simulink model "vestibular_system_final"  (Simulink 7.7)
settings: Solver=ode45  StartTime=0  StopTime=40  FixedStep=0.1
values from neighbouring files (symbols this model uses):
  a_lineal = get(hObject,'Value')-1    [interfaz_grafica.m]    (also in modelo_vestibular.m = 1)
  cabeza = get(hObject,'Value')-1    [interfaz_grafica.m]    (also in modelo_vestibular.m = 1)
  canal = get(hObject,'Value')-1    [interfaz_grafica.m]    (also in modelo_vestibular.m = 0)
  d = 0.76    [constantesvestibular.m]    (also in modelo_vestibular.m)
  eje_giro = get(hObject,'Value')-1    [interfaz_grafica.m]    (also in modelo_vestibular.m = 3)
  m = 1070    [constantesvestibular.m]    (also in modelo_vestibular.m)
  silla = get(hObject,'Value')-1    [interfaz_grafica.m]    (also in modelo_vestibular.m = 0)
  tau1 = 13.2    [constantesvestibular.m]    (also in modelo_vestibular.m)
  tau2 = 0.006    [constantesvestibular.m]    (also in modelo_vestibular.m)
undefined symbols (not defined in the file or in its folder): sigbuilder_block
settings Model: Creator=Ángel  LastModifiedBy=Ángel

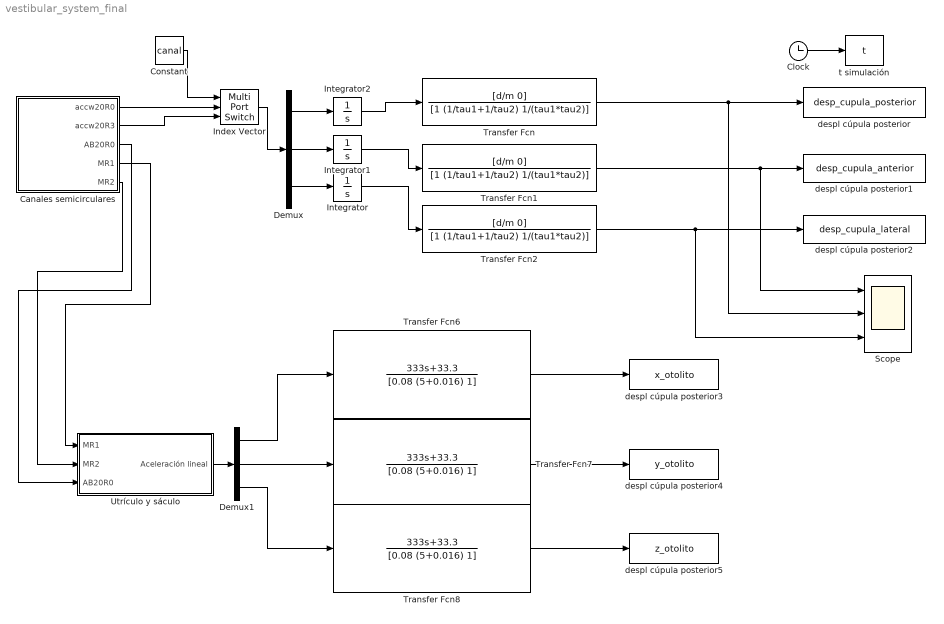
== system vestibular_system_final ==
  Canales semicirculares : Subsystem
  Clock : Clock
      settings: Decimation=10
  Constant : Constant  Value=canal
  Demux : Demux  Outputs=3
  Demux1 : Demux  Outputs=3
  Index Vector : MultiPortSwitch  DataPortOrder=Zero-based contiguous  Inputs=2  zeroidx=on
  Integrator : Integrator
  Integrator1 : Integrator
  Integrator2 : Integrator
  Scope : Scope  NumInputPorts=3
      settings: YMin=-5~-5~-5  YMax=5~5~5  SaveName=ScopeData6
  Transfer Fcn : TransferFcn  Numerator=[d/m 0]  Denominator=[1 (1/tau1+1/tau2) 1/(tau1*tau2)]
  Transfer Fcn1 : TransferFcn  Numerator=[d/m 0]  Denominator=[1 (1/tau1+1/tau2) 1/(tau1*tau2)]
  Transfer Fcn2 : TransferFcn  Numerator=[d/m 0]  Denominator=[1 (1/tau1+1/tau2) 1/(tau1*tau2)]
  Transfer Fcn6 : TransferFcn  Numerator=[333 33.3]  Denominator=[0.08 (5+0.016) 1]
  Transfer Fcn7 : TransferFcn  Numerator=[333 33.3]  Denominator=[0.08 (5+0.016) 1]
  Transfer Fcn8 : TransferFcn  Numerator=[333 33.3]  Denominator=[0.08 (5+0.016) 1]
  Utrículo y sáculo : Subsystem
  despl cúpula posterior : ToWorkspace  VariableName=desp_cupula_posterior  SampleTime=-1  SaveFormat=Array
  despl cúpula posterior1 : ToWorkspace  VariableName=desp_cupula_anterior  SampleTime=-1  SaveFormat=Array
  despl cúpula posterior2 : ToWorkspace  VariableName=desp_cupula_lateral  SampleTime=-1  SaveFormat=Array
  despl cúpula posterior3 : ToWorkspace  VariableName=x_otolito  SampleTime=-1  SaveFormat=Array
  despl cúpula posterior4 : ToWorkspace  VariableName=y_otolito  SampleTime=-1  SaveFormat=Array
  despl cúpula posterior5 : ToWorkspace  VariableName=z_otolito  SampleTime=-1  SaveFormat=Array
  t simulación : ToWorkspace  VariableName=t  SampleTime=-1  SaveFormat=Array
  wires:
  Constant/1 -> Index Vector/1
  Utrículo y sáculo/1(Aceleración lineal) -> Demux1/1
  Clock/1 -> t simulación/1
  Transfer Fcn/1 -> despl cúpula posterior/1, Scope/2
  Transfer Fcn1/1 -> despl cúpula posterior1/1, Scope/1
  Transfer Fcn2/1 -> despl cúpula posterior2/1, Scope/3
  Demux/1 -> Integrator2/1
  Demux/2 -> Integrator1/1
  Demux/3 -> Integrator/1
  Integrator2/1 -> Transfer Fcn/1
  Integrator1/1 -> Transfer Fcn1/1
  Integrator/1 -> Transfer Fcn2/1
  Canales semicirculares/1(accw20R0) -> Index Vector/2
  Canales semicirculares/2(accw20R3) -> Index Vector/3
  Canales semicirculares/3(AB20R0) -> Utrículo y sáculo/3(AB20R0)
  Canales semicirculares/4(MR1) -> Utrículo y sáculo/1(MR1)
  Canales semicirculares/5(MR2) -> Utrículo y sáculo/2(MR2)
  Index Vector/1 -> Demux/1
  Demux1/1 -> Transfer Fcn6/1
  Demux1/2 -> Transfer Fcn7/1
  Demux1/3 -> Transfer Fcn8/1
  Transfer Fcn6/1 -> despl cúpula posterior3/1
  Transfer Fcn7/1 -> despl cúpula posterior4/1
  Transfer Fcn8/1 -> despl cúpula posterior5/1

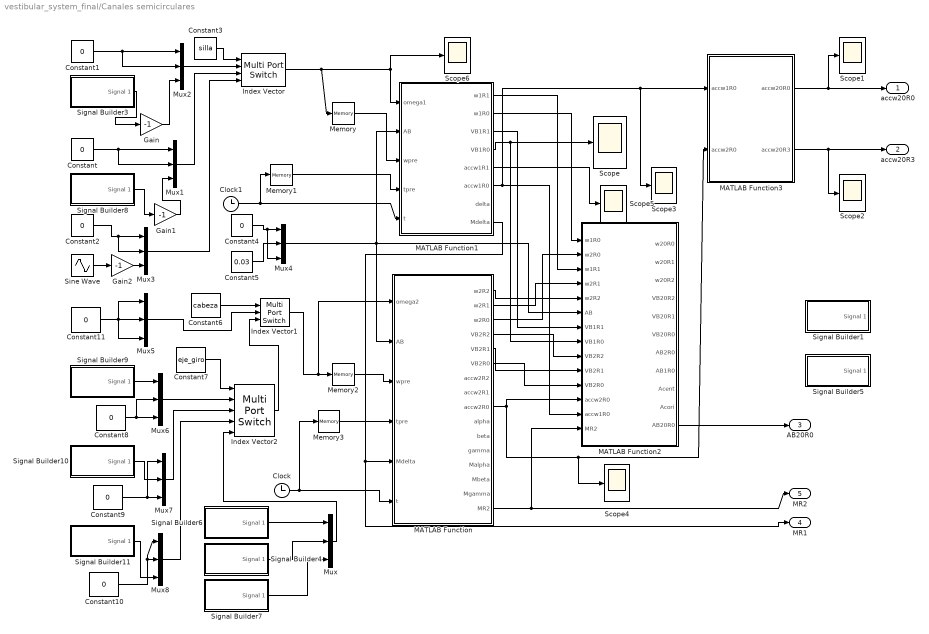
== system vestibular_system_final/Canales semicirculares ==
  Clock : Clock
      settings: Decimation=10
  Clock1 : Clock
      settings: Decimation=10
  Constant{,1..2,4,8..11} (8 alike) : Constant  Value=0
  Constant3 : Constant  Value=silla
  Constant5 : Constant  Value=0.03
  Constant6 : Constant  Value=cabeza
  Constant7 : Constant  Value=eje_giro
  Gain : Gain  Gain=-1
  Gain1 : Gain  Gain=-1
  Gain2 : Gain  Gain=-1
  Index Vector : MultiPortSwitch  DataPortOrder=Zero-based contiguous  zeroidx=on
  Index Vector1 : MultiPortSwitch  DataPortOrder=Zero-based contiguous  Inputs=2  zeroidx=on
  Index Vector2 : MultiPortSwitch  DataPortOrder=Zero-based contiguous  Inputs=4  zeroidx=on
  MATLAB Function : Stateflow chart  TreatAsAtomicUnit=on
  MATLAB Function1 : Stateflow chart  TreatAsAtomicUnit=on
  MATLAB Function2 : Stateflow chart  TreatAsAtomicUnit=on
  MATLAB Function3 : Stateflow chart  TreatAsAtomicUnit=on
  Memory{,1..3} (4 alike) : Memory
  Mux{,1..8} (9 alike) : Mux  Inputs=3
  Scope{,1..6} (7 alike) : Scope
      Scope2 settings: SaveName=ScopeData2
      Scope3 settings: SaveName=ScopeData3
      Scope4 settings: SaveName=ScopeData4
      Scope5 settings: TimeRange=40  YMin=0  YMax=0.16  SaveName=ScopeData7
      Scope6 settings: SaveName=ScopeData8
  Signal Builder1 : Subsystem  Tag=STV Subsys  LoadFcn=sigbuilder_block('load');  StartFcn=sigbuilder_block('start');  StopFcn=sigbuilder_block('stop');  ClipboardFcn=sigbuilder_block('clipboard');  mask(Sigbuilder block){}
      mask help: Create and generate interchangeable groups of signals whose waveforms are piecewise linear.
      mask init:
      | if ~strcmp(get_param(bdroot(gcbh),'SimulationStatus'),'stopped') tuvar = sigbuilder_block('maskInit'); end
      settings: CopyFcn=sigbuilder_block('copy');  DeleteFcn=sigbuilder_block('delete');  ModelCloseFcn=sigbuilder_block('modelClose');  PreSaveFcn=sigbuilder_block('preSave');  NameChangeFcn=sigbuilder_block('namechange');  OpenFcn=sigbuilder_block('open',[437.25 118.5 550.5 394.5 ]);  CloseFcn=sigbuilder_block('close');
      mask Display: plot(0, 0, 100, 100,[2, 2, 32, 32, 2], [68, 8, 8, 68, 68],[32, 2], [38, 38], [32, 19, 2],[53, 60, 44], [32, 17, 17, 2],[16, 16, 31, 31]);txt = getActiveGroup(gcbh);text(2, 100, txt,'verticalAlignment', 'top');
  Signal Builder10 : Subsystem  Tag=STV Subsys  LoadFcn=sigbuilder_block('load');  StartFcn=sigbuilder_block('start');  StopFcn=sigbuilder_block('stop');  ClipboardFcn=sigbuilder_block('clipboard');  mask(Sigbuilder block){}
      mask help: Create and generate interchangeable groups of signals whose waveforms are piecewise linear.
      mask init:
      | if ~strcmp(get_param(bdroot(gcbh),'SimulationStatus'),'stopped') tuvar = sigbuilder_block('maskInit'); end
      settings: CopyFcn=sigbuilder_block('copy');  DeleteFcn=sigbuilder_block('delete');  ModelCloseFcn=sigbuilder_block('modelClose');  PreSaveFcn=sigbuilder_block('preSave');  NameChangeFcn=sigbuilder_block('namechange');  OpenFcn=sigbuilder_block('open',[437.25 118.5 550.5 394.5 ]);  CloseFcn=sigbuilder_block('close');
      mask Display: plot(0, 0, 100, 100,[2, 2, 32, 32, 2], [68, 8, 8, 68, 68],[32, 2], [38, 38], [32, 19, 2],[53, 60, 44], [32, 17, 17, 2],[16, 16, 31, 31]);txt = getActiveGroup(gcbh);text(2, 100, txt,'verticalAlignment', 'top');
  Signal Builder11 : Subsystem  Tag=STV Subsys  LoadFcn=sigbuilder_block('load');  StartFcn=sigbuilder_block('start');  StopFcn=sigbuilder_block('stop');  ClipboardFcn=sigbuilder_block('clipboard');  mask(Sigbuilder block){}
      mask help: Create and generate interchangeable groups of signals whose waveforms are piecewise linear.
      mask init:
      | if ~strcmp(get_param(bdroot(gcbh),'SimulationStatus'),'stopped') tuvar = sigbuilder_block('maskInit'); end
      settings: CopyFcn=sigbuilder_block('copy');  DeleteFcn=sigbuilder_block('delete');  ModelCloseFcn=sigbuilder_block('modelClose');  PreSaveFcn=sigbuilder_block('preSave');  NameChangeFcn=sigbuilder_block('namechange');  OpenFcn=sigbuilder_block('open',[437.25 118.5 550.5 394.5 ]);  CloseFcn=sigbuilder_block('close');
      mask Display: plot(0, 0, 100, 100,[2, 2, 32, 32, 2], [68, 8, 8, 68, 68],[32, 2], [38, 38], [32, 19, 2],[53, 60, 44], [32, 17, 17, 2],[16, 16, 31, 31]);txt = getActiveGroup(gcbh);text(2, 100, txt,'verticalAlignment', 'top');
  Signal Builder3 : Subsystem  Tag=STV Subsys  LoadFcn=sigbuilder_block('load');  StartFcn=sigbuilder_block('start');  StopFcn=sigbuilder_block('stop');  ClipboardFcn=sigbuilder_block('clipboard');  mask(Sigbuilder block){}
      mask help: Create and generate interchangeable groups of signals whose waveforms are piecewise linear.
      mask init:
      | if ~strcmp(get_param(bdroot(gcbh),'SimulationStatus'),'stopped') tuvar = sigbuilder_block('maskInit'); end
      settings: CopyFcn=sigbuilder_block('copy');  DeleteFcn=sigbuilder_block('delete');  ModelCloseFcn=sigbuilder_block('modelClose');  PreSaveFcn=sigbuilder_block('preSave');  NameChangeFcn=sigbuilder_block('namechange');  OpenFcn=sigbuilder_block('open',[437.25 118.5 550.5 394.5 ]);  CloseFcn=sigbuilder_block('close');
      mask Display: plot(0, 0, 100, 100,[2, 2, 32, 32, 2], [68, 8, 8, 68, 68],[32, 2], [38, 38], [32, 19, 2],[53, 60, 44], [32, 17, 17, 2],[16, 16, 31, 31]);txt = getActiveGroup(gcbh);text(2, 100, txt,'verticalAlignment', 'top');
  Signal Builder4 : Subsystem  Tag=STV Subsys  LoadFcn=sigbuilder_block('load');  StartFcn=sigbuilder_block('start');  StopFcn=sigbuilder_block('stop');  ClipboardFcn=sigbuilder_block('clipboard');  mask(Sigbuilder block){}
      mask help: Create and generate interchangeable groups of signals whose waveforms are piecewise linear.
      mask init:
      | if ~strcmp(get_param(bdroot(gcbh),'SimulationStatus'),'stopped') tuvar = sigbuilder_block('maskInit'); end
      settings: CopyFcn=sigbuilder_block('copy');  DeleteFcn=sigbuilder_block('delete');  ModelCloseFcn=sigbuilder_block('modelClose');  PreSaveFcn=sigbuilder_block('preSave');  NameChangeFcn=sigbuilder_block('namechange');  OpenFcn=sigbuilder_block('open',[437.25 118.5 550.5 394.5 ]);  CloseFcn=sigbuilder_block('close');
      mask Display: plot(0, 0, 100, 100,[2, 2, 32, 32, 2], [68, 8, 8, 68, 68],[32, 2], [38, 38], [32, 19, 2],[53, 60, 44], [32, 17, 17, 2],[16, 16, 31, 31]);txt = getActiveGroup(gcbh);text(2, 100, txt,'verticalAlignment', 'top');
  Signal Builder5 : Subsystem  Tag=STV Subsys  LoadFcn=sigbuilder_block('load');  StartFcn=sigbuilder_block('start');  StopFcn=sigbuilder_block('stop');  ClipboardFcn=sigbuilder_block('clipboard');  mask(Sigbuilder block){}
      mask help: Create and generate interchangeable groups of signals whose waveforms are piecewise linear.
      mask init:
      | if ~strcmp(get_param(bdroot(gcbh),'SimulationStatus'),'stopped') tuvar = sigbuilder_block('maskInit'); end
      settings: CopyFcn=sigbuilder_block('copy');  DeleteFcn=sigbuilder_block('delete');  ModelCloseFcn=sigbuilder_block('modelClose');  PreSaveFcn=sigbuilder_block('preSave');  NameChangeFcn=sigbuilder_block('namechange');  OpenFcn=sigbuilder_block('open',[437.25 118.5 550.5 394.5 ]);  CloseFcn=sigbuilder_block('close');
      mask Display: plot(0, 0, 100, 100,[2, 2, 32, 32, 2], [68, 8, 8, 68, 68],[32, 2], [38, 38], [32, 19, 2],[53, 60, 44], [32, 17, 17, 2],[16, 16, 31, 31]);txt = getActiveGroup(gcbh);text(2, 100, txt,'verticalAlignment', 'top');
  Signal Builder6 : Subsystem  Tag=STV Subsys  LoadFcn=sigbuilder_block('load');  StartFcn=sigbuilder_block('start');  StopFcn=sigbuilder_block('stop');  ClipboardFcn=sigbuilder_block('clipboard');  mask(Sigbuilder block){}
      mask help: Create and generate interchangeable groups of signals whose waveforms are piecewise linear.
      mask init:
      | if ~strcmp(get_param(bdroot(gcbh),'SimulationStatus'),'stopped') tuvar = sigbuilder_block('maskInit'); end
      settings: CopyFcn=sigbuilder_block('copy');  DeleteFcn=sigbuilder_block('delete');  ModelCloseFcn=sigbuilder_block('modelClose');  PreSaveFcn=sigbuilder_block('preSave');  NameChangeFcn=sigbuilder_block('namechange');  OpenFcn=sigbuilder_block('open',[437.25 118.5 550.5 394.5 ]);  CloseFcn=sigbuilder_block('close');
      mask Display: plot(0, 0, 100, 100,[2, 2, 32, 32, 2], [68, 8, 8, 68, 68],[32, 2], [38, 38], [32, 19, 2],[53, 60, 44], [32, 17, 17, 2],[16, 16, 31, 31]);txt = getActiveGroup(gcbh);text(2, 100, txt,'verticalAlignment', 'top');
  Signal Builder7 : Subsystem  Tag=STV Subsys  LoadFcn=sigbuilder_block('load');  StartFcn=sigbuilder_block('start');  StopFcn=sigbuilder_block('stop');  ClipboardFcn=sigbuilder_block('clipboard');  mask(Sigbuilder block){}
      mask help: Create and generate interchangeable groups of signals whose waveforms are piecewise linear.
      mask init:
      | if ~strcmp(get_param(bdroot(gcbh),'SimulationStatus'),'stopped') tuvar = sigbuilder_block('maskInit'); end
      settings: CopyFcn=sigbuilder_block('copy');  DeleteFcn=sigbuilder_block('delete');  ModelCloseFcn=sigbuilder_block('modelClose');  PreSaveFcn=sigbuilder_block('preSave');  NameChangeFcn=sigbuilder_block('namechange');  OpenFcn=sigbuilder_block('open',[437.25 118.5 550.5 394.5 ]);  CloseFcn=sigbuilder_block('close');
      mask Display: plot(0, 0, 100, 100,[2, 2, 32, 32, 2], [68, 8, 8, 68, 68],[32, 2], [38, 38], [32, 19, 2],[53, 60, 44], [32, 17, 17, 2],[16, 16, 31, 31]);txt = getActiveGroup(gcbh);text(2, 100, txt,'verticalAlignment', 'top');
  Signal Builder8 : Subsystem  Tag=STV Subsys  LoadFcn=sigbuilder_block('load');  StartFcn=sigbuilder_block('start');  StopFcn=sigbuilder_block('stop');  ClipboardFcn=sigbuilder_block('clipboard');  mask(Sigbuilder block){}
      mask help: Create and generate interchangeable groups of signals whose waveforms are piecewise linear.
      mask init:
      | if ~strcmp(get_param(bdroot(gcbh),'SimulationStatus'),'stopped') tuvar = sigbuilder_block('maskInit'); end
      settings: CopyFcn=sigbuilder_block('copy');  DeleteFcn=sigbuilder_block('delete');  ModelCloseFcn=sigbuilder_block('modelClose');  PreSaveFcn=sigbuilder_block('preSave');  NameChangeFcn=sigbuilder_block('namechange');  OpenFcn=sigbuilder_block('open',[437.25 118.5 550.5 394.5 ]);  CloseFcn=sigbuilder_block('close');
      mask Display: plot(0, 0, 100, 100,[2, 2, 32, 32, 2], [68, 8, 8, 68, 68],[32, 2], [38, 38], [32, 19, 2],[53, 60, 44], [32, 17, 17, 2],[16, 16, 31, 31]);txt = getActiveGroup(gcbh);text(2, 100, txt,'verticalAlignment', 'top');
  Signal Builder9 : Subsystem  Tag=STV Subsys  LoadFcn=sigbuilder_block('load');  StartFcn=sigbuilder_block('start');  StopFcn=sigbuilder_block('stop');  ClipboardFcn=sigbuilder_block('clipboard');  mask(Sigbuilder block){}
      mask help: Create and generate interchangeable groups of signals whose waveforms are piecewise linear.
      mask init:
      | if ~strcmp(get_param(bdroot(gcbh),'SimulationStatus'),'stopped') tuvar = sigbuilder_block('maskInit'); end
      settings: CopyFcn=sigbuilder_block('copy');  DeleteFcn=sigbuilder_block('delete');  ModelCloseFcn=sigbuilder_block('modelClose');  PreSaveFcn=sigbuilder_block('preSave');  NameChangeFcn=sigbuilder_block('namechange');  OpenFcn=sigbuilder_block('open',[437.25 118.5 550.5 394.5 ]);  CloseFcn=sigbuilder_block('close');
      mask Display: plot(0, 0, 100, 100,[2, 2, 32, 32, 2], [68, 8, 8, 68, 68],[32, 2], [38, 38], [32, 19, 2],[53, 60, 44], [32, 17, 17, 2],[16, 16, 31, 31]);txt = getActiveGroup(gcbh);text(2, 100, txt,'verticalAlignment', 'top');
  Sine Wave : Sin  Amplitude=1.7453  Frequency=0.5  SampleTime=0
  accw20R0 : Outport
  accw20R3 : Outport  Port=2
  AB20R0 : Outport  Port=3
  MR1 : Outport  Port=4
  MR2 : Outport  Port=5
  wires:
  MATLAB Function/16(MR2) -> MATLAB Function2/14(MR2), MR2/1
  Clock/1 -> Memory3/1, MATLAB Function/6(t)
  Constant/1 -> Mux1/1, Mux1/2
  Constant1/1 -> Mux2/1, Mux2/2
  Constant2/1 -> Mux3/1, Mux3/2
  Constant3/1 -> Index Vector/1
  Mux3/1 -> Index Vector/4
  Constant4/1 -> Mux4/1, Mux4/3
  Constant5/1 -> Mux4/2
  Mux4/1 -> MATLAB Function1/2(AB), MATLAB Function/2(AB), MATLAB Function2/6(AB)
  Index Vector/1 -> Memory/1, MATLAB Function1/1(omega1), Scope6/1
  Clock1/1 -> MATLAB Function1/5(t), Memory1/1
  MATLAB Function1/4(VB1R0) -> Scope/1, MATLAB Function2/8(VB1R0)
  MATLAB Function1/8(Mdelta) -> MATLAB Function/5(Mdelta), MR1/1
  MATLAB Function/3(w2R0) -> MATLAB Function2/2(w2R0)
  MATLAB Function1/2(w1R0) -> MATLAB Function2/1(w1R0)
  MATLAB Function1/1(w1R1) -> MATLAB Function2/3(w1R1)
  MATLAB Function/2(w2R1) -> MATLAB Function2/4(w2R1)
  MATLAB Function/1(w2R2) -> MATLAB Function2/5(w2R2)
  MATLAB Function/4(VB2R2) -> MATLAB Function2/9(VB2R2)
  MATLAB Function/5(VB2R1) -> MATLAB Function2/10(VB2R1)
  MATLAB Function/6(VB2R0) -> MATLAB Function2/11(VB2R0)
  MATLAB Function1/3(VB1R1) -> MATLAB Function2/7(VB1R1)
  MATLAB Function1/6(accw1R0) -> MATLAB Function3/1(accw1R0), Scope3/1, MATLAB Function2/13(accw1R0)
  MATLAB Function/9(accw2R0) -> MATLAB Function3/2(accw2R0), Scope4/1, MATLAB Function2/12(accw2R0)
  MATLAB Function3/2(accw20R3) -> Scope2/1, accw20R3/1
  MATLAB Function2/11(AB20R0) -> AB20R0/1
  MATLAB Function3/1(accw20R0) -> Scope1/1, accw20R0/1
  MATLAB Function1/5(accw1R1) -> Scope5/1
  Memory1/1 -> MATLAB Function1/4(tpre)
  Memory/1 -> MATLAB Function1/3(wpre)
  Memory2/1 -> MATLAB Function/3(wpre)
  Memory3/1 -> MATLAB Function/4(tpre)
  Gain/1 -> Mux2/3
  Constant11/1 -> Mux5/2, Mux5/3, Mux5/1
  Signal Builder4/1(Signal 1) -> Mux/2
  Index Vector1/1 -> Memory2/1, MATLAB Function/1(omega2)
  Constant6/1 -> Index Vector1/1
  Signal Builder7/1(Signal 1) -> Mux/3
  Signal Builder6/1(Signal 1) -> Mux/1
  Mux2/1 -> Index Vector/2
  Mux1/1 -> Index Vector/3
  Constant7/1 -> Index Vector2/1
  Signal Builder9/1(Signal 1) -> Mux6/1
  Constant8/1 -> Mux6/2, Mux6/3
  Mux6/1 -> Index Vector2/2
  Mux7/1 -> Index Vector2/3
  Mux8/1 -> Index Vector2/4
  Mux5/1 -> Index Vector1/2
  Index Vector2/1 -> Index Vector1/3
  Signal Builder10/1(Signal 1) -> Mux7/2
  Constant9/1 -> Mux7/3, Mux7/1
  Signal Builder11/1(Signal 1) -> Mux8/3
  Constant10/1 -> Mux8/1, Mux8/2
  Mux/1 -> Index Vector2/5
  Signal Builder8/1(Signal 1) -> Gain1/1
  Gain1/1 -> Mux1/3
  Signal Builder3/1(Signal 1) -> Gain/1
  Sine Wave/1 -> Gain2/1
  Gain2/1 -> Mux3/3

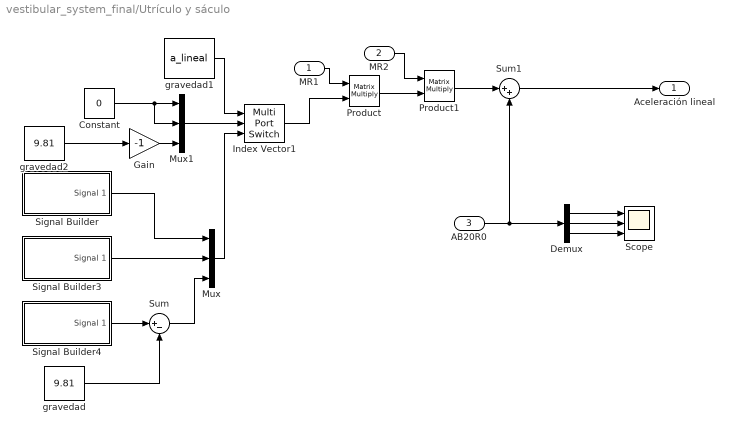
== system vestibular_system_final/Utrículo y sáculo ==
  MR1 : Inport
  MR2 : Inport  Port=2
  AB20R0 : Inport  Port=3
  Constant : Constant  Value=0
  Demux : Demux  Outputs=3
  Gain : Gain  Gain=-1
  Index Vector1 : MultiPortSwitch  DataPortOrder=Zero-based contiguous  Inputs=2  zeroidx=on
  Mux : Mux  Inputs=3
  Mux1 : Mux  Inputs=3
  Product : Product  Multiplication=Matrix(*)  RndMeth=Zero
  Product1 : Product  Multiplication=Matrix(*)  RndMeth=Zero
  Scope : Scope  NumInputPorts=3
      settings: YMin=-5~-5~-5  YMax=5~5~5  SaveName=ScopeData5
  Signal Builder : Subsystem  Tag=STV Subsys  LoadFcn=sigbuilder_block('load');  StartFcn=sigbuilder_block('start');  StopFcn=sigbuilder_block('stop');  ClipboardFcn=sigbuilder_block('clipboard');  mask(Sigbuilder block){}
      mask help: Create and generate interchangeable groups of signals whose waveforms are piecewise linear.
      mask init:
      | if ~strcmp(get_param(bdroot(gcbh),'SimulationStatus'),'stopped') tuvar = sigbuilder_block('maskInit'); end
      settings: CopyFcn=sigbuilder_block('copy');  DeleteFcn=sigbuilder_block('delete');  ModelCloseFcn=sigbuilder_block('modelClose');  PreSaveFcn=sigbuilder_block('preSave');  NameChangeFcn=sigbuilder_block('namechange');  OpenFcn=sigbuilder_block('open',[437.25 118.5 550.5 394.5 ]);  CloseFcn=sigbuilder_block('close');
      mask Display: plot(0, 0, 100, 100,[2, 2, 32, 32, 2], [68, 8, 8, 68, 68],[32, 2], [38, 38], [32, 19, 2],[53, 60, 44], [32, 17, 17, 2],[16, 16, 31, 31]);txt = getActiveGroup(gcbh);text(2, 100, txt,'verticalAlignment', 'top');
  Signal Builder3 : Subsystem  Tag=STV Subsys  LoadFcn=sigbuilder_block('load');  StartFcn=sigbuilder_block('start');  StopFcn=sigbuilder_block('stop');  ClipboardFcn=sigbuilder_block('clipboard');  mask(Sigbuilder block){}
      mask help: Create and generate interchangeable groups of signals whose waveforms are piecewise linear.
      mask init:
      | if ~strcmp(get_param(bdroot(gcbh),'SimulationStatus'),'stopped') tuvar = sigbuilder_block('maskInit'); end
      settings: CopyFcn=sigbuilder_block('copy');  DeleteFcn=sigbuilder_block('delete');  ModelCloseFcn=sigbuilder_block('modelClose');  PreSaveFcn=sigbuilder_block('preSave');  NameChangeFcn=sigbuilder_block('namechange');  OpenFcn=sigbuilder_block('open',[437.25 118.5 550.5 394.5 ]);  CloseFcn=sigbuilder_block('close');
      mask Display: plot(0, 0, 100, 100,[2, 2, 32, 32, 2], [68, 8, 8, 68, 68],[32, 2], [38, 38], [32, 19, 2],[53, 60, 44], [32, 17, 17, 2],[16, 16, 31, 31]);txt = getActiveGroup(gcbh);text(2, 100, txt,'verticalAlignment', 'top');
  Signal Builder4 : Subsystem  Tag=STV Subsys  LoadFcn=sigbuilder_block('load');  StartFcn=sigbuilder_block('start');  StopFcn=sigbuilder_block('stop');  ClipboardFcn=sigbuilder_block('clipboard');  mask(Sigbuilder block){}
      mask help: Create and generate interchangeable groups of signals whose waveforms are piecewise linear.
      mask init:
      | if ~strcmp(get_param(bdroot(gcbh),'SimulationStatus'),'stopped') tuvar = sigbuilder_block('maskInit'); end
      settings: CopyFcn=sigbuilder_block('copy');  DeleteFcn=sigbuilder_block('delete');  ModelCloseFcn=sigbuilder_block('modelClose');  PreSaveFcn=sigbuilder_block('preSave');  NameChangeFcn=sigbuilder_block('namechange');  OpenFcn=sigbuilder_block('open',[437.25 118.5 550.5 394.5 ]);  CloseFcn=sigbuilder_block('close');
      mask Display: plot(0, 0, 100, 100,[2, 2, 32, 32, 2], [68, 8, 8, 68, 68],[32, 2], [38, 38], [32, 19, 2],[53, 60, 44], [32, 17, 17, 2],[16, 16, 31, 31]);txt = getActiveGroup(gcbh);text(2, 100, txt,'verticalAlignment', 'top');
  Sum : Sum  Inputs=|+-
  Sum1 : Sum  Inputs=|++
  gravedad : Constant  Value=9.81
  gravedad1 : Constant  Value=a_lineal
  gravedad2 : Constant  Value=9.81
  Aceleración lineal : Outport
  wires:
  Signal Builder/1(Signal 1) -> Mux/1
  Sum/1 -> Mux/3
  gravedad/1 -> Sum/2
  Product/1 -> Product1/2
  Product1/1 -> Sum1/1
  AB20R0/1 -> Sum1/2, Demux/1
  MR1/1 -> Product/1
  MR2/1 -> Product1/1
  Demux/1 -> Scope/1
  Demux/2 -> Scope/2
  Demux/3 -> Scope/3
  Signal Builder3/1(Signal 1) -> Mux/2
  Signal Builder4/1(Signal 1) -> Sum/1
  Sum1/1 -> Aceleración lineal/1
  Index Vector1/1 -> Product/2
  Mux/1 -> Index Vector1/3
  gravedad1/1 -> Index Vector1/1
  Mux1/1 -> Index Vector1/2
  Constant/1 -> Mux1/2, Mux1/1
  gravedad2/1 -> Gain/1
  Gain/1 -> Mux1/3

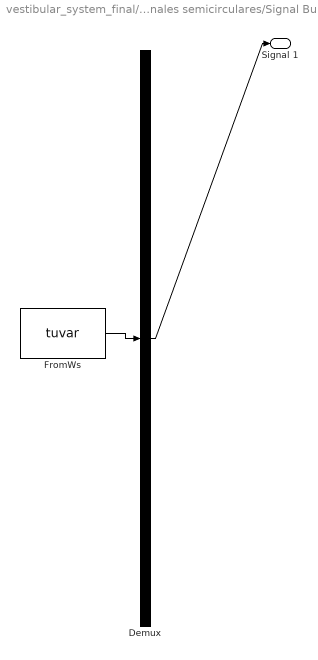
== system vestibular_system_final/Canales semicirculares/Signal Builder1 ==
  Demux : Demux  Tag=STV Demux  Outputs=1
  FromWs : FromWorkspace  Tag=STV FromWs  VariableName=tuvar  SampleTime=0  SigBuilderData=DataTag0  VnvData=DataTag1
      SigBuilderData=|
      | common.afterFinalStr = 'Extrapolate'
      | common.sampleTime = 0
      | dataSet.timeRange = [0 40]
      | dataSet.name = 'Group 1'
      | sbobj.Groups.Name = 'Group 1'
      | sbobj.Groups.Signals.Name = 'Signal 1'
      | sbobj.Groups.Signals.XData = [0 10 10.7 24 25 25.7 39 40]
      | sbobj.Groups.Signals.YData = [0 0 0.9 0.9 0 -0.9 -0.9 0]
      | sbobj.Groups.TimeRange = [0 40]
  Signal 1 : Outport  Tag=STV Outport
  wires:
  FromWs/1 -> Demux/1
  Demux/1 -> Signal 1/1

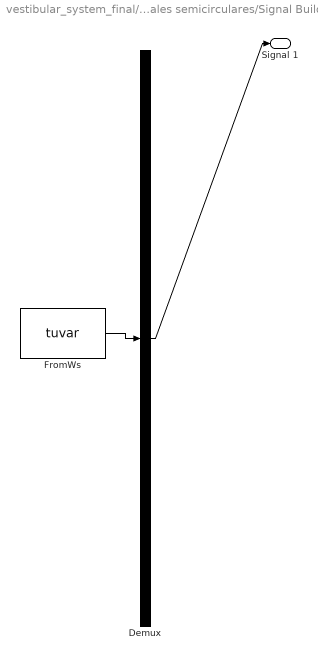
== system vestibular_system_final/Canales semicirculares/Signal Builder10 ==
  Demux : Demux  Tag=STV Demux  Outputs=1
  FromWs : FromWorkspace  Tag=STV FromWs  VariableName=tuvar  SampleTime=0  SigBuilderData=DataTag2  VnvData=DataTag3
      SigBuilderData=|
      | common.afterFinalStr = 'Extrapolate'
      | common.sampleTime = 0
      | dataSet.timeRange = [0 40]
      | dataSet.name = 'Group 1'
      | sbobj.Groups.Name = 'Group 1'
      | sbobj.Groups.Signals.Name = 'Signal 1'
      | sbobj.Groups.Signals.XData = [0 10 10.7 11 25 25.7 26 40]
      | sbobj.Groups.Signals.YData = [0 0 1.57079632679 0 0 -1.57079632679 0 0]
      | sbobj.Groups.TimeRange = [0 40]
  Signal 1 : Outport  Tag=STV Outport
  wires:
  Demux/1 -> Signal 1/1
  FromWs/1 -> Demux/1

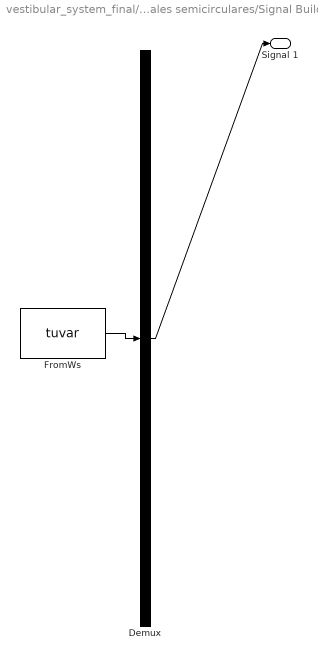
== system vestibular_system_final/Canales semicirculares/Signal Builder11 ==
  Demux : Demux  Tag=STV Demux  Outputs=1
  FromWs : FromWorkspace  Tag=STV FromWs  VariableName=tuvar  SampleTime=0  SigBuilderData=DataTag4  VnvData=DataTag5
      SigBuilderData=|
      | common.afterFinalStr = 'Extrapolate'
      | common.sampleTime = 0
      | dataSet.timeRange = [0 40]
      | dataSet.name = 'Group 1'
      | sbobj.Groups.Name = 'Group 1'
      | sbobj.Groups.Signals.Name = 'Signal 1'
      | sbobj.Groups.Signals.XData = [0 10 10.7 25 25.7 39 40]
      | sbobj.Groups.Signals.YData = [0 0 0.9 0 -0.9 -0.9 0]
      | sbobj.Groups.TimeRange = [0 40]
  Signal 1 : Outport  Tag=STV Outport
  wires:
  FromWs/1 -> Demux/1
  Demux/1 -> Signal 1/1

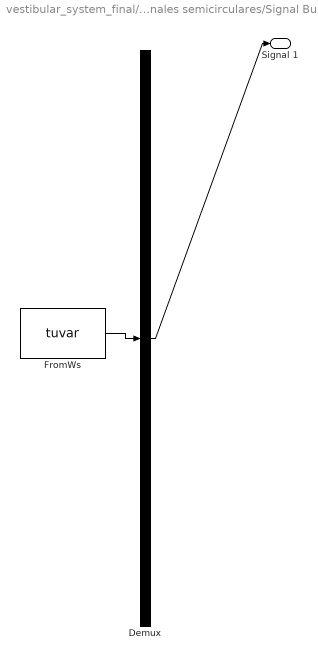
== system vestibular_system_final/Canales semicirculares/Signal Builder3 ==
  Demux : Demux  Tag=STV Demux  Outputs=1
  FromWs : FromWorkspace  Tag=STV FromWs  VariableName=tuvar  SampleTime=0  SigBuilderData=DataTag6  VnvData=DataTag7
      SigBuilderData=|
      | common.afterFinalStr = 'Extrapolate'
      | common.sampleTime = 0
      | dataSet.timeRange = [0 40]
      | dataSet.name = 'Group 1'
      | sbobj.Groups.Name = 'Group 1'
      | sbobj.Groups.Signals.Name = 'Signal 1'
      | sbobj.Groups.Signals.XData = [0 0.98 1 2 8 10 40]
      | sbobj.Groups.Signals.YData = [0 0 0 1.74532925199 1.74532925199 1.74532925199 1.74532925199]
      | sbobj.Groups.TimeRange = [0 40]
  Signal 1 : Outport  Tag=STV Outport
  wires:
  Demux/1 -> Signal 1/1
  FromWs/1 -> Demux/1

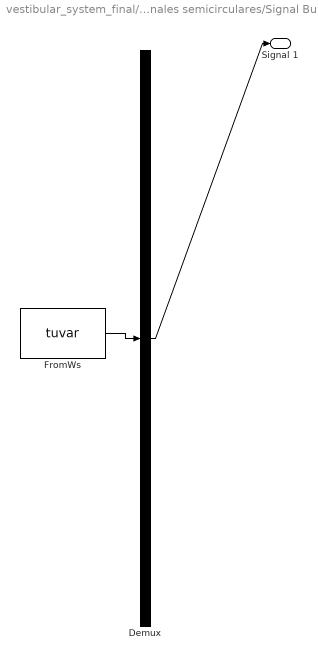
== system vestibular_system_final/Canales semicirculares/Signal Builder4 ==
  Demux : Demux  Tag=STV Demux  Outputs=1
  FromWs : FromWorkspace  Tag=STV FromWs  VariableName=tuvar  SampleTime=0  SigBuilderData=DataTag8  VnvData=DataTag9
      SigBuilderData=|
      | common.afterFinalStr = 'Extrapolate'
      | common.sampleTime = 0
      | dataSet.timeRange = [0 40]
      | dataSet.name = 'Group 1'
      | sbobj.Groups.Name = 'Group 1'
      | sbobj.Groups.Signals.Name = 'Signal 1'
      | sbobj.Groups.Signals.XData = [0 10 10.7 11 25 25.7 26 40]
      | sbobj.Groups.Signals.YData = [0 0 1.57079632679 0 0 -1.57079632679 0 0]
      | sbobj.Groups.TimeRange = [0 40]
  Signal 1 : Outport  Tag=STV Outport
  wires:
  FromWs/1 -> Demux/1
  Demux/1 -> Signal 1/1

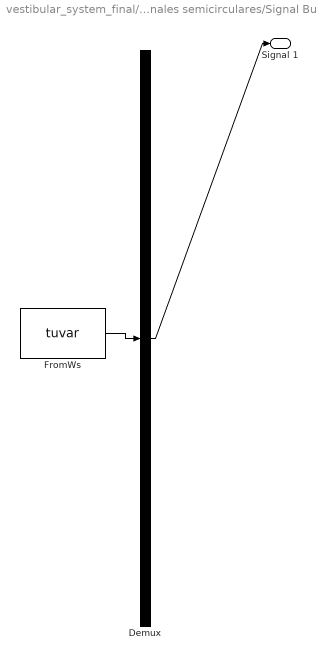
== system vestibular_system_final/Canales semicirculares/Signal Builder5 ==
  Demux : Demux  Tag=STV Demux  Outputs=1
  FromWs : FromWorkspace  Tag=STV FromWs  VariableName=tuvar  SampleTime=0  SigBuilderData=DataTag10  VnvData=DataTag11
      SigBuilderData=|
      | common.afterFinalStr = 'Extrapolate'
      | common.sampleTime = 0
      | dataSet.timeRange = [0 40]
      | dataSet.name = 'Group 1'
      | sbobj.Groups.Name = 'Group 1'
      | sbobj.Groups.Signals.Name = 'Signal 1'
      | sbobj.Groups.Signals.XData = [0 10 10.7 25 25.7 40]
      | sbobj.Groups.Signals.YData = [0 0 0.9 0 -0.9 0]
      | sbobj.Groups.TimeRange = [0 40]
  Signal 1 : Outport  Tag=STV Outport
  wires:
  Demux/1 -> Signal 1/1
  FromWs/1 -> Demux/1

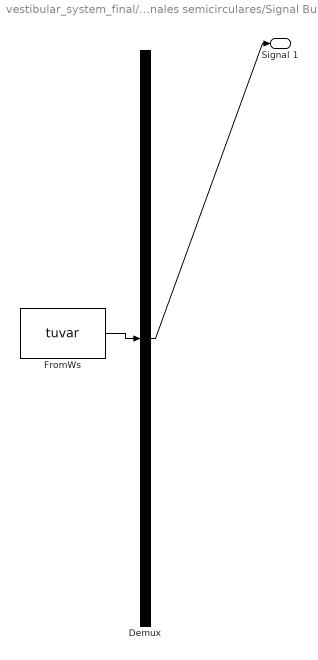
== system vestibular_system_final/Canales semicirculares/Signal Builder6 ==
  Demux : Demux  Tag=STV Demux  Outputs=1
  FromWs : FromWorkspace  Tag=STV FromWs  VariableName=tuvar  SampleTime=0  SigBuilderData=DataTag12  VnvData=DataTag13
      SigBuilderData=|
      | common.afterFinalStr = 'Extrapolate'
      | common.sampleTime = 0
      | dataSet.timeRange = [0 40]
      | dataSet.name = 'Group 1'
      | sbobj.Groups.Name = 'Group 1'
      | sbobj.Groups.Signals.Name = 'Signal 1'
      | sbobj.Groups.Signals.XData = [0 10 10.7 25 25.7 39 40]
      | sbobj.Groups.Signals.YData = [0 0 0.9 0 -0.9 -0.9 0]
      | sbobj.Groups.TimeRange = [0 40]
  Signal 1 : Outport  Tag=STV Outport
  wires:
  FromWs/1 -> Demux/1
  Demux/1 -> Signal 1/1

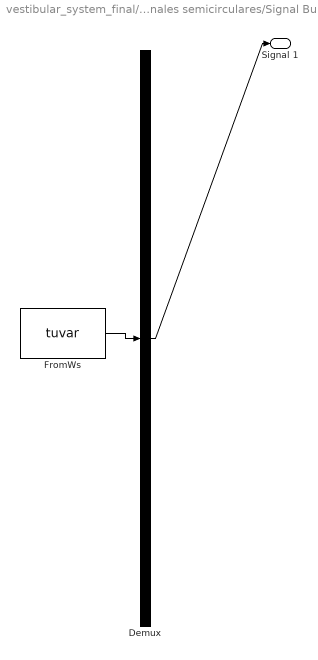
== system vestibular_system_final/Canales semicirculares/Signal Builder7 ==
  Demux : Demux  Tag=STV Demux  Outputs=1
  FromWs : FromWorkspace  Tag=STV FromWs  VariableName=tuvar  SampleTime=0  SigBuilderData=DataTag14  VnvData=DataTag15
      SigBuilderData=|
      | common.afterFinalStr = 'Extrapolate'
      | common.sampleTime = 0
      | dataSet.timeRange = [0 40]
      | dataSet.name = 'Group 1'
      | sbobj.Groups.Name = 'Group 1'
      | sbobj.Groups.Signals.Name = 'Signal 1'
      | sbobj.Groups.Signals.XData = [0 10 10.7 25 25.7 39 40]
      | sbobj.Groups.Signals.YData = [0 0 0.9 0 -0.9 -0.9 0]
      | sbobj.Groups.TimeRange = [0 40]
  Signal 1 : Outport  Tag=STV Outport
  wires:
  Demux/1 -> Signal 1/1
  FromWs/1 -> Demux/1

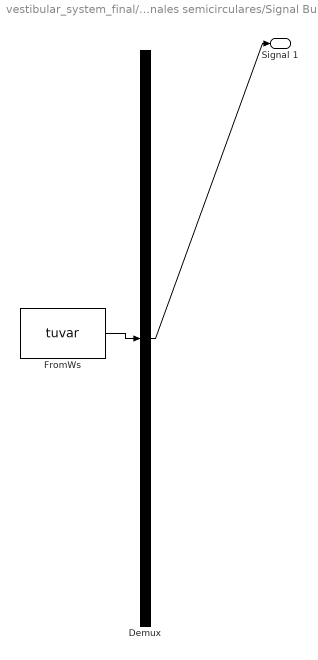
== system vestibular_system_final/Canales semicirculares/Signal Builder8 ==
  Demux : Demux  Tag=STV Demux  Outputs=1
  FromWs : FromWorkspace  Tag=STV FromWs  VariableName=tuvar  SampleTime=0  SigBuilderData=DataTag16  VnvData=DataTag17
      SigBuilderData=|
      | common.afterFinalStr = 'Extrapolate'
      | common.sampleTime = 0
      | dataSet.timeRange = [0 40]
      | dataSet.name = 'Group 1'
      | sbobj.Groups.Name = 'Group 1'
      | sbobj.Groups.Signals.Name = 'Signal 1'
      | sbobj.Groups.Signals.XData = [0 1 3 20 22 40]
      | sbobj.Groups.Signals.YData = [0 0 1.74532925199 1.74532925199 0 0]
      | sbobj.Groups.TimeRange = [0 40]
  Signal 1 : Outport  Tag=STV Outport
  wires:
  FromWs/1 -> Demux/1
  Demux/1 -> Signal 1/1

== system vestibular_system_final/Canales semicirculares/Signal Builder9 ==
  Demux : Demux  Tag=STV Demux  Outputs=1
  FromWs : FromWorkspace  Tag=STV FromWs  VariableName=tuvar  SampleTime=0  SigBuilderData=DataTag18  VnvData=DataTag19
      SigBuilderData=|
      | common.afterFinalStr = 'Extrapolate'
      | common.sampleTime = 0
      | dataSet.timeRange = [0 40]
      | dataSet.name = 'Group 1'
      | sbobj.Groups.Name = 'Group 1'
      | sbobj.Groups.Signals.Name = 'Signal 1'
      | sbobj.Groups.Signals.XData = [0 10 10.7 25 25.7 39 40]
      | sbobj.Groups.Signals.YData = [0 0 0.9 0 -0.9 -0.9 0]
      | sbobj.Groups.TimeRange = [0 40]
  Signal 1 : Outport  Tag=STV Outport
  wires:
  Demux/1 -> Signal 1/1
  FromWs/1 -> Demux/1

== system vestibular_system_final/Utrículo y sáculo/Signal Builder ==
  Demux : Demux  Tag=STV Demux  Outputs=1
  FromWs : FromWorkspace  Tag=STV FromWs  VariableName=tuvar  SampleTime=0  SigBuilderData=DataTag20  VnvData=DataTag21
      SigBuilderData=|
      | common.afterFinalStr = 'Extrapolate'
      | common.sampleTime = 0
      | dataSet.timeRange = [0 10]
      | dataSet.name = 'Group 1'
      | sbobj.Groups.Name = 'Group 1'
      | sbobj.Groups.Signals.Name = 'Signal 1'
      | sbobj.Groups.Signals.XData = [0 3 4 6 7 10]
      | sbobj.Groups.Signals.YData = [0 0 1 1 0 0]
  Signal 1 : Outport  Tag=STV Outport
  wires:
  Demux/1 -> Signal 1/1
  FromWs/1 -> Demux/1

== system vestibular_system_final/Utrículo y sáculo/Signal Builder3 ==
  Demux : Demux  Tag=STV Demux  Outputs=1
  FromWs : FromWorkspace  Tag=STV FromWs  VariableName=tuvar  SampleTime=0  SigBuilderData=DataTag22  VnvData=DataTag23
      SigBuilderData=|
      | common.afterFinalStr = 'Extrapolate'
      | common.sampleTime = 0
      | dataSet.timeRange = [0 10]
      | dataSet.name = 'Group 1'
      | sbobj.Groups.Name = 'Group 1'
      | sbobj.Groups.Signals.Name = 'Signal 1'
      | sbobj.Groups.Signals.XData = [0 3 4 6 7 10]
      | sbobj.Groups.Signals.YData = [0 0 1 1 0 0]
  Signal 1 : Outport  Tag=STV Outport
  wires:
  FromWs/1 -> Demux/1
  Demux/1 -> Signal 1/1

== system vestibular_system_final/Utrículo y sáculo/Signal Builder4 ==
  Demux : Demux  Tag=STV Demux  Outputs=1
  FromWs : FromWorkspace  Tag=STV FromWs  VariableName=tuvar  SampleTime=0  SigBuilderData=DataTag24  VnvData=DataTag25
      SigBuilderData=|
      | common.afterFinalStr = 'Extrapolate'
      | common.sampleTime = 0
      | dataSet.timeRange = [0 10]
      | dataSet.name = 'Group 1'
      | sbobj.Groups.Name = 'Group 1'
      | sbobj.Groups.Signals.Name = 'Signal 1'
      | sbobj.Groups.Signals.XData = [0 3 4 6 7 10]
      | sbobj.Groups.Signals.YData = [0 0 1 1 0 0]
  Signal 1 : Outport  Tag=STV Outport
  wires:
  Demux/1 -> Signal 1/1
  FromWs/1 -> Demux/1

== matlab function Canales semicirculares/MATLAB Function1 ==
  data: w1R1 output double; w1R0 output double; omega1 input double; AB input double; wpre input double; tpre input double; t input double; VB1R1 output double; VB1R0 output double; accw1R1 output double; accw1R0 output double; delta output double; Mdelta output double
function [w1R1,w1R0,VB1R1,VB1R0,accw1R1,accw1R0,delta,Mdelta]= fcn(omega1,AB,wpre,tpre,t)
%#codegen
%velocidad angular de la silla (rad/s) en R2
%w1R2 = MR2*omega1;

%velocidad angular de la silla (rad/s) en R1
w1R1 = omega1;

%ángulo delta de la silla respecto al sistema R0
%delta = int(omega1(3),0,t); ángulo recorrido por la silla si la vel
%angular es una función
delta = omega1(3)*(t-tpre); %ángulo recorrido por la silla si la vel
%angular es un valor numérico

Mdelta=[cos(delta) sin(delta) 0; -sin(delta) cos(delta) 0; 0 0 1];

%velocidad angular de la silla (rad/s) en R0
w1R0 = Mdelta*omega1;

%aceleración angular de la silla en R1
%w1acc = [0 0 0]; para velocidad constante de la silla
%accw1R1 = diff(omega1(3),t); aceleración angular si tuvieramos una función
%de la velocidad 
% Aceleración angular de la silla en R1
if t == 0
  accw1R1 = [0; 0; 0];  
else    
    accw1R1 = (omega1-wpre)/(t-tpre); % aceleración angular si tenemos un valor numérico de la velocidad angular    
end
% Aceleración angular de la silla en R0
accw1R0 = Mdelta*accw1R1;

%velocidad lineal del punto B en R1 debido a la velocidad de la silla
VB1R1 = cross(w1R1,AB);

%velocidad lineal de la silla en R0 debido a la velocidad de la silla
VB1R0 = cross(w1R0,AB);

== matlab function Canales semicirculares/MATLAB Function ==
  data: w2R2 output double; omega2 input double; AB input double; wpre input double; tpre input double; Mdelta input double; t input double; w2R1 output double; w2R0 output double; VB2R2 output double; VB2R1 output double; VB2R0 output double; accw2R2 output double; accw2R1 output double; accw2R0 output double; alpha output double; beta output double; gamma output double; Malpha output double; Mbeta output double; Mgamma output double; MR2 output double
function [w2R2,w2R1,w2R0,VB2R2,VB2R1,VB2R0,accw2R2,accw2R1,accw2R0,alpha,beta,gamma,Malpha,Mbeta,Mgamma,MR2] = fcn(omega2,AB,wpre,tpre,Mdelta,t)
%#codegen

%velocidad angular de la cabeza (los 3 ejes) en R2
w2R2 = omega2;

%ángulo roll
alpha = omega2(1)*(t-tpre);

%ángulo pitch
beta = omega2(2)*(t-tpre);

%ángulo yaw
gamma = omega2(3)*(t-tpre);

%matrices de cambio de sistema de referencia
Malpha = [1 0 0; 0 cos(alpha) sin(alpha); 0 -sin(alpha) cos(alpha)];
Mbeta = [cos(beta) 0 -sin(beta); 0 1 0; sin(beta) 0 cos(beta)];
Mgamma = [cos(gamma) sin(gamma) 0; -sin(gamma) cos(gamma) 0; 0 0 1];
MR2 = Malpha*Mbeta*Mgamma;

%velocidad angular de la cabeza en R1
w2R1 = Malpha*Mbeta*Mgamma*omega2;

%velocidad angular de la cabeza en R0
w2R0 = Malpha*Mbeta*Mgamma*Mdelta*omega2;

% Aceleración angular de la cabeza en R2
if t == 0
    accw2R2 = [0; 0; 0];
else    
    accw2R2 = (omega2-wpre)/(t-tpre);
end    

% Aceleración angular de la cabeza en R1
accw2R1 = MR2*accw2R2;

% Aceleración angular de la cabeza en R0
accw2R0 = MR2*Mdelta*accw2R2;

%velocidad lineal del punto B en R2 debido a la velocidad de la cabeza
VB2R2 = cross(w2R2,AB);

%velocidad lineal del punto B en R1 debido a la velocidad de la cabeza
VB2R1 = cross(w2R1,AB);

%velocidad lineal del punto B en R0 debido a la velocidad de la cabeza
VB2R0 = cross(w2R0,AB);

== matlab function Canales semicirculares/MATLAB Function2 ==
  data: w1R0 input double; w20R0 output double; w2R0 input double; w1R1 input double; w2R1 input double; w2R2 input double; AB input double; VB1R1 input double; VB1R0 input double; VB2R2 input double; VB2R1 input double; VB2R0 input double; accw2R0 input double; accw1R0 input double; w20R1 output double; w20R2 output double; MR2 input double; VB20R2 output double; VB20R1 output double; VB20R0 output double; AB2R0 output double; AB1R0 output double; Acent output double; Acori output double; AB20R0 output double
function [w20R0,w20R1,w20R2,VB20R2,VB20R1,VB20R0,AB2R0,AB1R0,Acent,Acori,AB20R0]= fcn(w1R0,w2R0,w1R1,w2R1,w2R2,AB,VB1R1,VB1R0,VB2R2,VB2R1,VB2R0,accw2R0,accw1R0,MR2)
%#codegen

% Velocidad angular de la contribución silla+cabeza en el sistema de referencia earth (R0)
w20R0 = w2R0+w1R0;

% Velocidad angular de la contribución silla+cabeza en R1
w20R1 = w2R1+w1R1;

% Velocidad angular de la contribución silla+cabeza en R2
w1R2 = MR2*w1R1;
w20R2 = w2R2+w1R2;

% velocidad lineal del punto B en R2 debido a la velocidad de la cabeza +
% silla
VB1R2 = cross(w1R2,AB);
VB20R2 = VB2R2+VB1R2;

% velocidad lineal del punto B en R1 debido a la velocidad de la cabeza +
% silla
VB20R1 = VB2R1+VB1R1;

% velocidad lineal del punto B en R0 debido a la velocidad de la cabeza +
% silla
VB20R0 = VB2R0+VB1R0;

% Aceleraciones lienales (4 términos)
% primer término
AB2R0 = cross(accw2R0,AB);

% segundo término
AB1R0 = cross(accw1R0,AB);

% tercer término (aceleración centrípeta)
Acent = cross(w1R0,cross(w1R0,AB));

% cuarto término (aceleración de coriolis)
Acori = 2*cross(w1R0,VB2R0);

% Aceleración absoluta
AB20R0 = AB2R0+AB1R0+Acent+Acori;

== matlab function Canales semicirculares/MATLAB Function3 ==
  data: accw1R0 input double; accw20R0 output double; accw20R3 output double; accw2R0 input double
function [accw20R0,accw20R3] = fcn(accw1R0,accw2R0)
%#codegen

% Aceleración angular de la contribución silla+cabeza en el sistema earth
% (R0)
accw20R0 = accw2R0+accw1R0;

% ángulos de Euler canales semicirculares (rad)

chia=2.212;
chip=2.336;
chil=0;
thetaa=0.177;
thetap=0;
thetal=-0.331;
fia=0;
fip=-0.274;
fil=0.038;

%matriz de trasformación a R3

MR3=[cos(thetaa)*cos(chia) cos(thetaa)*sin(chia) -sin(thetaa); -cos(fip)*sin(chip) cos(fip)*cos(chip) sin(fip); cos(fil)*sin(thetal) -sin(fil) cos(fil)*cos(thetal)];

% Aceleración angular de la contribución silla+cabeza en el sistema de los
% canales semicirculares (R3)
% accw20R3 = (MR3*accw2R0)+(MR3*accw1R0);

accw20R3 = MR3*accw20R0;
